simulink model "Tank"  (Simulink 7.7)
settings: Solver=ode45  StartTime=0.0  StopTime=10.0  RelTol=1e-3
settings Model: Creator=Owner  LastModifiedBy=Owner

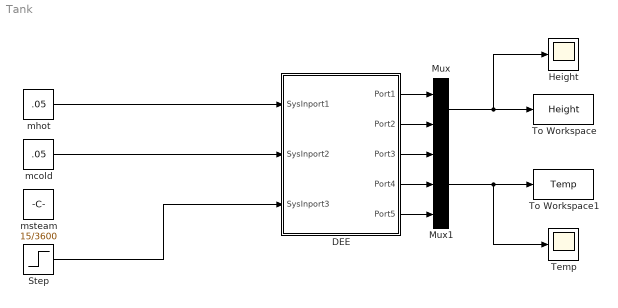
== system Tank ==
  DEE : Subsystem
      settings: OpenFcn=diffeqed
      mask Type: Differential Equation Editor (DEE)
      mask Display: disp('Heated Tank in Series')
  Height : Scope
  Mux : Mux  Inputs=2
  Mux1 : Mux  Inputs=3
  Step : Step  Before=15/3600  After=15/3600*.95  SampleTime=0
  Temp : Scope
  To Workspace : ToWorkspace  VariableName=Height  SampleTime=-1  SaveFormat=Structure
  To Workspace1 : ToWorkspace  VariableName=Temp  SampleTime=-1  SaveFormat=Structure
  mcold : Constant  Value=.05
  mhot : Constant  Value=.05
  msteam : Constant  Value=15/3600
  wires:
  DEE/1(Port1) -> Mux/1
  DEE/2(Port2) -> Mux/2
  DEE/3(Port3) -> Mux1/1
  DEE/4(Port4) -> Mux1/2
  DEE/5(Port5) -> Mux1/3
  Mux/1 -> To Workspace/1, Height/1
  Mux1/1 -> To Workspace1/1, Temp/1
  mhot/1 -> DEE/1(SysInport1)
  mcold/1 -> DEE/2(SysInport2)
  Step/1 -> DEE/3(SysInport3)

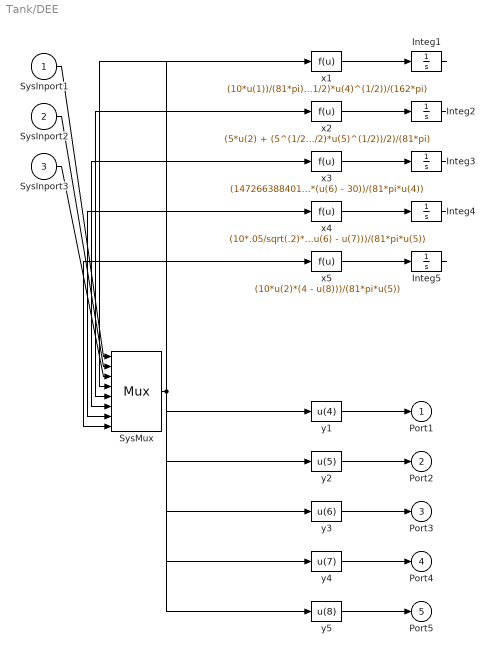
== system Tank/DEE ==
  SysInport1 : Inport
  SysInport2 : Inport  Port=2
  SysInport3 : Inport  Port=3
  Integ1 : Integrator  InitialCondition=.2
  Integ2 : Integrator  InitialCondition=.2
  Integ3 : Integrator  InitialCondition=70
  Integ4 : Integrator  InitialCondition=70
  Integ5 : Integrator  InitialCondition=4
  SysMux : Mux  Inputs=8
  x1 : Fcn  Expr=(10*u(1))/(81*pi) - (5^(1/2)*u(4)^(1/2))/(162*pi)
  x2 : Fcn  Expr=(5*u(2) + (5^(1/2)*u(4)^(1/2))/4 - (5^(1/2)*u(5)^(1/2))/2)/(81*pi)
  x3 : Fcn  Expr=(147266388401061888*u(3))/(7807119111329159*u(4)) - (10*u(1)*(u(6) - 30))/(81*pi*u(4))
  x4 : Fcn  Expr=(10*.05/sqrt(.2)*u(4)^(1/2)*(u(6) - u(7)))/(81*pi*u(5))
  x5 : Fcn  Expr=(10*u(2)*(4 - u(8)))/(81*pi*u(5))
  y1 : Fcn  Expr=u(4)
  y2 : Fcn  Expr=u(5)
  y3 : Fcn  Expr=u(6)
  y4 : Fcn  Expr=u(7)
  y5 : Fcn  Expr=u(8)
  Port1 : Outport
  Port2 : Outport  Port=2
  Port3 : Outport  Port=3
  Port4 : Outport  Port=4
  Port5 : Outport  Port=5
  wires:
  SysInport1/1 -> SysMux/1
  SysInport2/1 -> SysMux/2
  SysInport3/1 -> SysMux/3
  SysMux/1 -> x1/1, x2/1, x3/1, x4/1, x5/1, y1/1, y2/1, y3/1, y4/1, y5/1
  x1/1 -> Integ1/1
  Integ1/1 -> SysMux/4
  x2/1 -> Integ2/1
  Integ2/1 -> SysMux/5
  x3/1 -> Integ3/1
  Integ3/1 -> SysMux/6
  x4/1 -> Integ4/1
  Integ4/1 -> SysMux/7
  x5/1 -> Integ5/1
  Integ5/1 -> SysMux/8
  y1/1 -> Port1/1
  y2/1 -> Port2/1
  y3/1 -> Port3/1
  y4/1 -> Port4/1
  y5/1 -> Port5/1
